simulink model "full_adder"  (R2020a)
settings: Solver=VariableStepAuto  StartTime=0.0  StopTime=10  RelTol=1e-3
settings Model: Creator=F1  LastModifiedBy=F1

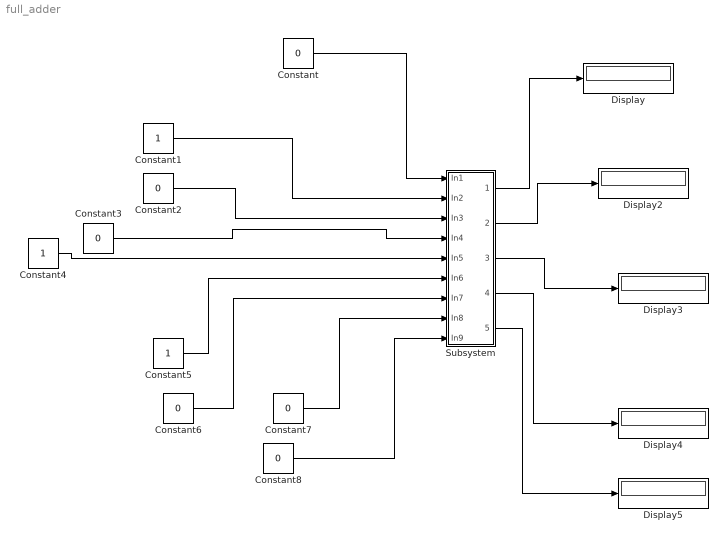
== system full_adder ==
  Constant{,2..3,6..8} (6 alike) : Constant  Value=0
  Constant1 : Constant
  Constant4 : Constant
  Constant5 : Constant
  Display{,2..5} (5 alike) : Display
  Subsystem : Subsystem
  wires:
  Constant/1 -> Subsystem/1(In1)
  Constant1/1 -> Subsystem/2(In2)
  Constant2/1 -> Subsystem/3(In3)
  Constant3/1 -> Subsystem/4(In4)
  Constant4/1 -> Subsystem/5(In5)
  Constant5/1 -> Subsystem/6(In6)
  Constant6/1 -> Subsystem/7(In7)
  Constant7/1 -> Subsystem/8(In8)
  Constant8/1 -> Subsystem/9(In9)
  Subsystem/1(Out1) -> Display/1
  Subsystem/2(Out2) -> Display2/1
  Subsystem/3(Out3) -> Display3/1
  Subsystem/4(Out4) -> Display4/1
  Subsystem/5(Out5) -> Display5/1

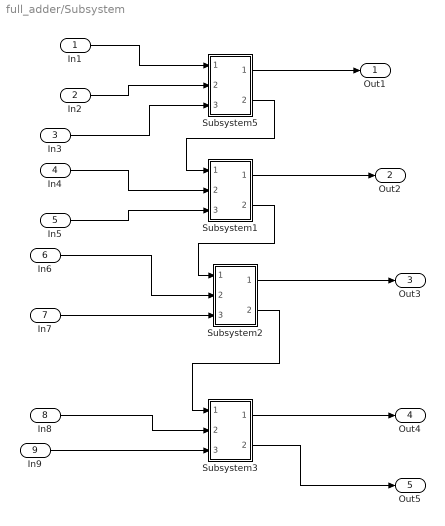
== system full_adder/Subsystem ==
  In1 : Inport
  In2 : Inport  Port=2
  In3 : Inport  Port=3
  In4 : Inport  Port=4
  In5 : Inport  Port=5
  In6 : Inport  Port=6
  In7 : Inport  Port=7
  In8 : Inport  Port=8
  In9 : Inport  Port=9
  Subsystem1 : Subsystem
  Subsystem2 : Subsystem
  Subsystem3 : Subsystem
  Subsystem5 : Subsystem
  Out1 : Outport
  Out2 : Outport  Port=2
  Out3 : Outport  Port=3
  Out4 : Outport  Port=4
  Out5 : Outport  Port=5
  wires:
  Subsystem2/2(Out2) -> Subsystem3/1(In1)
  In8/1 -> Subsystem3/2(In2)
  Subsystem5/2(Out2) -> Subsystem1/1(In1)
  Subsystem2/1(Out1) -> Out3/1
  Subsystem1/2(Out2) -> Subsystem2/1(In1)
  In6/1 -> Subsystem2/2(In2)
  In7/1 -> Subsystem2/3(In3)
  In4/1 -> Subsystem1/2(In2)
  Subsystem3/1(Out1) -> Out4/1
  In9/1 -> Subsystem3/3(In3)
  In2/1 -> Subsystem5/2(In2)
  In3/1 -> Subsystem5/3(In3)
  In1/1 -> Subsystem5/1(In1)
  Subsystem5/1(Out1) -> Out1/1
  Subsystem3/2(Out2) -> Out5/1
  Subsystem1/1(Out1) -> Out2/1
  In5/1 -> Subsystem1/3(In3)

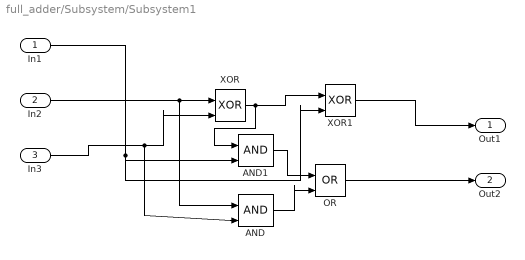
== system full_adder/Subsystem/Subsystem1 ==
  In1 : Inport
  In2 : Inport  Port=2
  In3 : Inport  Port=3
  AND : Logic  IconShape=distinctive  AllPortsSameDT=off  OutDataTypeStr=boolean
  AND1 : Logic  IconShape=distinctive  AllPortsSameDT=off  OutDataTypeStr=boolean
  OR : Logic  Operator=OR  IconShape=distinctive  AllPortsSameDT=off  OutDataTypeStr=boolean
  XOR : Logic  Operator=XOR  IconShape=distinctive  AllPortsSameDT=off  OutDataTypeStr=boolean
  XOR1 : Logic  Operator=XOR  IconShape=distinctive  AllPortsSameDT=off  OutDataTypeStr=boolean
  Out1 : Outport
  Out2 : Outport  Port=2
  wires:
  AND1/1 -> OR/1
  AND/1 -> OR/2
  In3/1 -> AND/2, XOR/2
  In2/1 -> AND/1, XOR/1
  In1/1 -> XOR1/2, AND1/2
  XOR/1 -> AND1/1, XOR1/1
  XOR1/1 -> Out1/1
  OR/1 -> Out2/1

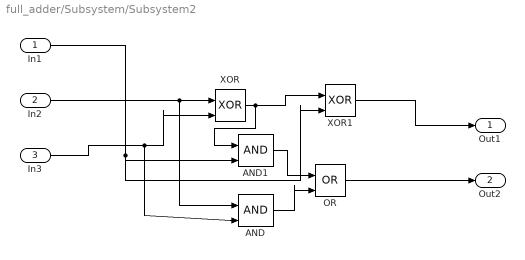
== system full_adder/Subsystem/Subsystem2 ==
  In1 : Inport
  In2 : Inport  Port=2
  In3 : Inport  Port=3
  AND : Logic  IconShape=distinctive  AllPortsSameDT=off  OutDataTypeStr=boolean
  AND1 : Logic  IconShape=distinctive  AllPortsSameDT=off  OutDataTypeStr=boolean
  OR : Logic  Operator=OR  IconShape=distinctive  AllPortsSameDT=off  OutDataTypeStr=boolean
  XOR : Logic  Operator=XOR  IconShape=distinctive  AllPortsSameDT=off  OutDataTypeStr=boolean
  XOR1 : Logic  Operator=XOR  IconShape=distinctive  AllPortsSameDT=off  OutDataTypeStr=boolean
  Out1 : Outport
  Out2 : Outport  Port=2
  wires:
  AND1/1 -> OR/1
  AND/1 -> OR/2
  In3/1 -> AND/2, XOR/2
  In2/1 -> AND/1, XOR/1
  In1/1 -> XOR1/2, AND1/2
  XOR/1 -> AND1/1, XOR1/1
  XOR1/1 -> Out1/1
  OR/1 -> Out2/1

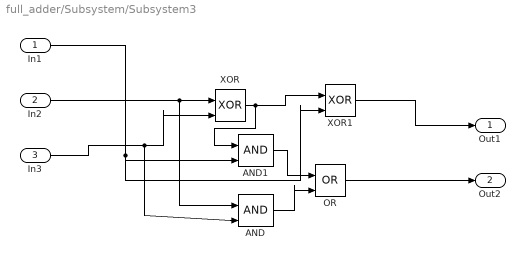
== system full_adder/Subsystem/Subsystem3 ==
  In1 : Inport
  In2 : Inport  Port=2
  In3 : Inport  Port=3
  AND : Logic  IconShape=distinctive  AllPortsSameDT=off  OutDataTypeStr=boolean
  AND1 : Logic  IconShape=distinctive  AllPortsSameDT=off  OutDataTypeStr=boolean
  OR : Logic  Operator=OR  IconShape=distinctive  AllPortsSameDT=off  OutDataTypeStr=boolean
  XOR : Logic  Operator=XOR  IconShape=distinctive  AllPortsSameDT=off  OutDataTypeStr=boolean
  XOR1 : Logic  Operator=XOR  IconShape=distinctive  AllPortsSameDT=off  OutDataTypeStr=boolean
  Out1 : Outport
  Out2 : Outport  Port=2
  wires:
  AND1/1 -> OR/1
  AND/1 -> OR/2
  In3/1 -> AND/2, XOR/2
  In2/1 -> AND/1, XOR/1
  In1/1 -> XOR1/2, AND1/2
  XOR/1 -> AND1/1, XOR1/1
  XOR1/1 -> Out1/1
  OR/1 -> Out2/1

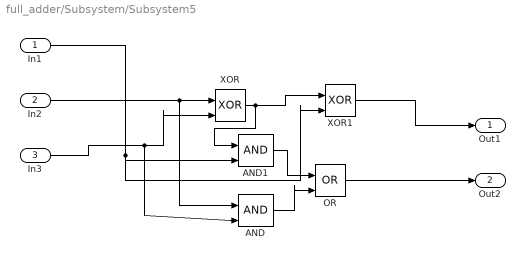
== system full_adder/Subsystem/Subsystem5 ==
  In1 : Inport
  In2 : Inport  Port=2
  In3 : Inport  Port=3
  AND : Logic  IconShape=distinctive  AllPortsSameDT=off  OutDataTypeStr=boolean
  AND1 : Logic  IconShape=distinctive  AllPortsSameDT=off  OutDataTypeStr=boolean
  OR : Logic  Operator=OR  IconShape=distinctive  AllPortsSameDT=off  OutDataTypeStr=boolean
  XOR : Logic  Operator=XOR  IconShape=distinctive  AllPortsSameDT=off  OutDataTypeStr=boolean
  XOR1 : Logic  Operator=XOR  IconShape=distinctive  AllPortsSameDT=off  OutDataTypeStr=boolean
  Out1 : Outport
  Out2 : Outport  Port=2
  wires:
  AND1/1 -> OR/1
  AND/1 -> OR/2
  In3/1 -> AND/2, XOR/2
  In2/1 -> AND/1, XOR/1
  In1/1 -> XOR1/2, AND1/2
  XOR/1 -> AND1/1, XOR1/1
  XOR1/1 -> Out1/1
  OR/1 -> Out2/1
